simulink model "Controlador"  (Simulink 7.3)
settings: Solver=ode45  StartTime=0.0  StopTime=100  MaxStep=0.03  MinStep=0.01  RelTol=1e-3
values from neighbouring files (symbols this model uses):
  K = lqr(A,B,Q,R)    [LQR.m]    (also in bestQ.m = setK_lqr(Q_i); graficosPenduloReal.m = setK_lqr(Q_optimo))
libraries: simulink x2
settings Model: Creator=Daniel  LastModifiedBy=Daniel
settings SolverCC: InitialStep=0.01

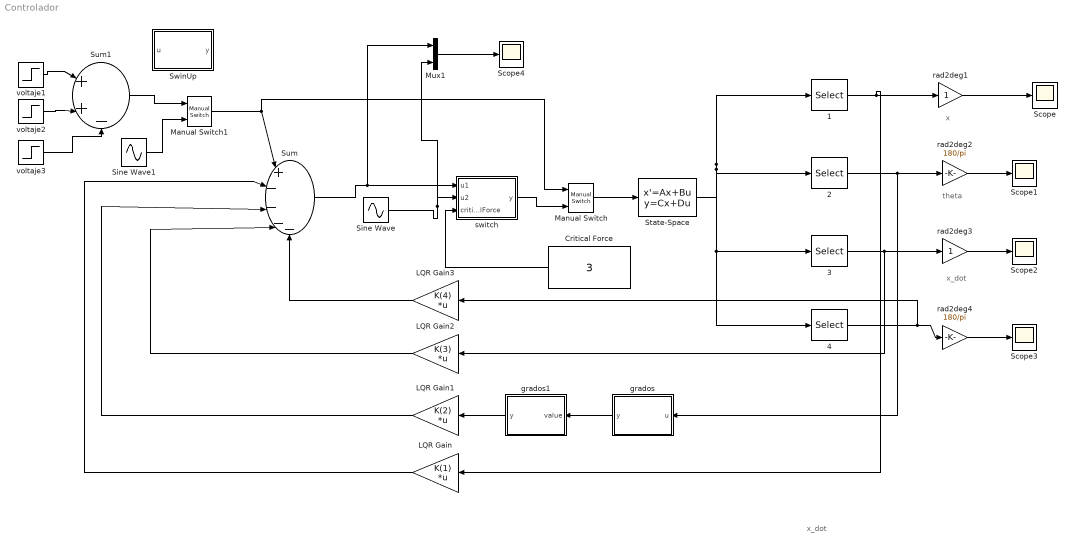
== system Controlador ==
  note: x
  note: theta
  note: x_dot
  note: x_dot
  " 1" : Selector  InputPortWidth=4  IndexOptions=Index vector (dialog)  Indices=1  OutputSizes=1
  " 2" : Selector  InputPortWidth=4  IndexOptions=Index vector (dialog)  Indices=2  OutputSizes=1
  " 3" : Selector  InputPortWidth=4  IndexOptions=Index vector (dialog)  Indices=3  OutputSizes=1
  " 4" : Selector  InputPortWidth=4  IndexOptions=Index vector (dialog)  Indices=4  OutputSizes=1
  Critical Force : Constant  Value=3  OutDataType=fixdt(1, 16)  OutScaling=2^0
  LQR Gain : Gain  Gain=K(1)  Multiplication=Matrix(K*u)  SaturateOnIntegerOverflow=on  OutDataTypeStr=Inherit: Same as input  ParamDataTypeStr=Inherit: Same as input
  LQR Gain1 : Gain  Gain=K(2)  Multiplication=Matrix(K*u)  SaturateOnIntegerOverflow=on  OutDataTypeStr=Inherit: Same as input  ParamDataTypeStr=Inherit: Same as input
  LQR Gain2 : Gain  Gain=K(3)  Multiplication=Matrix(K*u)  SaturateOnIntegerOverflow=on  OutDataTypeStr=Inherit: Same as input  ParamDataTypeStr=Inherit: Same as input
  LQR Gain3 : Gain  Gain=K(4)  Multiplication=Matrix(K*u)  SaturateOnIntegerOverflow=on  OutDataTypeStr=Inherit: Same as input  ParamDataTypeStr=Inherit: Same as input
  Manual Switch : simulink/Signal Routing/Manual Switch  SystemSampleTime=-1  sw=0  action=0  varsize=off
  Manual Switch1 : simulink/Signal Routing/Manual Switch  SystemSampleTime=-1  sw=0  action=0  varsize=off
  Mux1 : Mux  Inputs=2
  Scope{,1..4} (5 alike) : Scope
      Scope2 settings: SaveName=ScopeData2
      Scope3 settings: SaveName=ScopeData3
      Scope4 settings: SaveName=ScopeData4
  Sine Wave : Sin  Amplitude=5  Bias=0  Frequency=1  Phase=0  Samples=10  SampleTime=0  Offset=0
  Sine Wave1 : Sin  Amplitude=5  Bias=0  Frequency=0.05  Phase=0  Samples=10  SampleTime=0.1  Offset=0
  State-Space : StateSpace  A="[0 0 1 0; 0 0 0 1; 0 0.5401 -0.7235 0; 0  14.955 -0.9854 0]"  B="[0  ;0 ;2.2747 ;3.0978]"  C=eye(4)  D=[0;0;0;0]  X0=[ 0 ; 0i; 0; 0 ]
  Sum : Sum  Inputs=|+----  OutDataType=fixdt(1, 16)  OutScaling=2^0
  Sum1 : Sum  Inputs=|++-  OutDataType=fixdt(1, 16)  OutScaling=2^0
  SwinUp : Stateflow chart
  grados : Stateflow chart
  grados1 : Stateflow chart
  rad2deg1 : Gain  SaturateOnIntegerOverflow=on  OutDataTypeStr=Inherit: Same as input  ParamDataTypeStr=Inherit: Same as input
  rad2deg2 : Gain  Gain=180/pi  SaturateOnIntegerOverflow=on  OutDataTypeStr=Inherit: Same as input  ParamDataTypeStr=Inherit: Same as input
  rad2deg3 : Gain  SaturateOnIntegerOverflow=on  OutDataTypeStr=Inherit: Same as input  ParamDataTypeStr=Inherit: Same as input
  rad2deg4 : Gain  Gain=180/pi  SaturateOnIntegerOverflow=on  OutDataTypeStr=Inherit: Same as input  ParamDataTypeStr=Inherit: Same as input
  switch : Stateflow chart
  voltaje1 : Step  Time=20  After=3  SampleTime=0
  voltaje2 : Step  Time=50  After=2  SampleTime=0
  voltaje3 : Step  Time=80  SampleTime=0
  wires:
  " 1"/1 -> rad2deg1/1, LQR Gain/1
  " 2"/1 -> rad2deg2/1, grados/1(u)
  " 3"/1 -> rad2deg3/1, LQR Gain2/1
  rad2deg4/1 -> Scope3/1
  rad2deg3/1 -> Scope2/1
  rad2deg2/1 -> Scope1/1
  LQR Gain/1 -> Sum/2
  LQR Gain1/1 -> Sum/3
  LQR Gain2/1 -> Sum/4
  LQR Gain3/1 -> Sum/5
  State-Space/1 -> " 1"/1, " 2"/1, " 3"/1, " 4"/1
  " 4"/1 -> rad2deg4/1, LQR Gain3/1
  Sum/1 -> Mux1/1, switch/1(u1)
  Sine Wave/1 -> switch/2(u2), Mux1/2
  Critical Force/1 -> switch/3(criticalForce)
  rad2deg1/1 -> Scope/1
  Mux1/1 -> Scope4/1
  Manual Switch/1 -> State-Space/1
  switch/1(y) -> Manual Switch/2
  grados1/1(y) -> LQR Gain1/1
  grados/1(y) -> grados1/1(value)
  voltaje1/1 -> Sum1/1
  voltaje2/1 -> Sum1/2
  voltaje3/1 -> Sum1/3
  Sum1/1 -> Manual Switch1/1
  Sine Wave1/1 -> Manual Switch1/2
  Manual Switch1/1 -> Sum/1, Manual Switch/1

== matlab function switch ==
  data: u1 input double; y output double; u2 input double; criticalForce input double
function y = fcn(u1,u2,criticalForce)
%#eml

if (abs(u2) < criticalForce) 
    y = u1;
else
    y = u1;
end

== matlab function SwinUp ==
  data: u input double; y output double
function y = fcn(u)
%#eml
%y = sin(u);
y=exp(u)*sin(10*u);
end

== matlab function grados ==
  data: u input double; y output double
function y = fcn(u)
%#codegen

    y = mod(u,2*pi);
end

== matlab function grados1 ==
  data: value input double; y output double
function y = remapRange(value)
    scaleFactor = pi/180;
    if (value>180*scaleFactor)
        %constants
        fromLow = 181*scaleFactor;
        fromHigh = 360*scaleFactor;
        toLow = -179*scaleFactor;
        toHigh = 0*scaleFactor;
        %calculations
        new_range = toHigh-toLow;
        old_range = fromHigh - fromLow;
        new_value = (new_range/old_range)*(value-fromLow)+toLow;
        y = new_value;
    else
        y = value;
    end
        
end
